simulink model "One_D_admittance_simulink"  (R2019b)
settings: Solver=ode45  StartTime=0.0  StopTime=50.0  RelTol=1e-4
model workspace (MAT data in the model file):
  k = Simulink.Parameter
  k.DataType = 'auto'
  k.Dimensions = [0 0]
  k_p = -0.125
libraries: simulink x1
settings Model: OrderedModelArguments=off  Creator=KEYUR  LastModifiedBy=KEYUR
settings DataIOCC: ExternalInput=[t, y]  InitialState=initi_x  LoadExternalInput=on

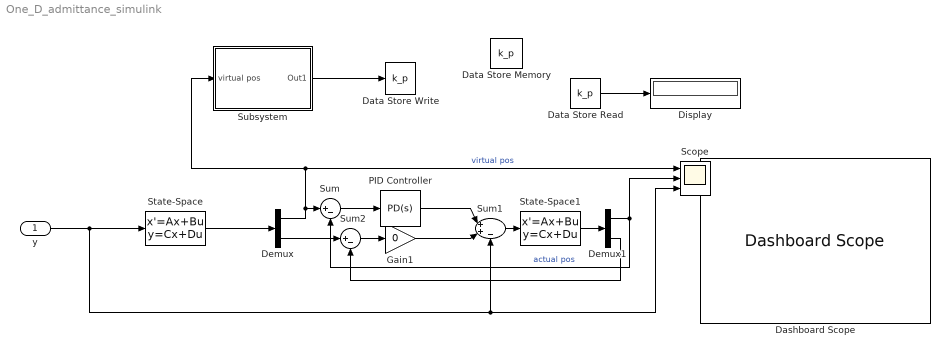
== system One_D_admittance_simulink ==
  y : Inport
  Dashboard Scope : DashboardScope  LegendPosition=Right
  Data Store Read : DataStoreRead  DataStoreName=k_p
  Data Store Write : DataStoreWrite  DataStoreName=k_p  DataStoreElements=k_p
  Data Store Memory : DataStoreMemory  DataStoreName=k_p  ReadBeforeWriteMsg=warning  WriteAfterWriteMsg=warning  WriteAfterReadMsg=warning  InitialValue=-10/40  VectorParams1D=off  ShowAdditionalParam=off  OutDataTypeStr=double
  Demux : Demux  Outputs=2
  Demux1 : Demux  Outputs=2
  Display : Display
  Gain1 : Gain  Gain=0
  PID Controller : simulink/Continuous/PID Controller  Controller=PD  Form=Parallel  TimeDomain=Continuous-time  SampleTime=-1  IntegratorMethod=Forward Euler  FilterMethod=Forward Euler  ControllerParametersSource=internal  P=85.3147223046163  I=6.85461887395414  D=89.8142135829374  UseFilter=on  N=224.237663795174  TunerSelectOption=Transfer Function Based (PID Tuner App)  InitialConditionSource=internal  InitialConditionForIntegrator=0  InitialConditionForFilter=0  DifferentiatorICPrevScaledInput=0  ExternalReset=none  TrackingMode=off  Kt=1  LimitOutput=off  UpperSaturationLimit=inf  LowerSaturationLimit=-inf  LinearizeAsGain=on  AntiWindupMode=none  Kb=1  POutMin=[]  POutMax=[]  IOutMin=[]  IOutMax=[]  DOutMin=[]  DOutMax=[]  NOutMin=[]  NOutMax=[]  SumOutMin=[]  SumOutMax=[]  SaturationOutMin=[]  SaturationOutMax=[]  PParamMin=[]  PParamMax=[]  IParamMin=[]  IParamMax=[]  DParamMin=[]  DParamMax=[]  NParamMin=[]  NParamMax=[]  KbParamMin=[]  KbParamMax=[]  KtParamMin=[]  KtParamMax=[]  KbOutMin=[]  KbOutMax=[]  KtOutMin=[]  KtOutMax=[]  IntegratorOutMin=[]  IntegratorOutMax=[]  FilterOutMin=[]  FilterOutMax=[]  SumI1OutMin=[]  SumI1OutMax=[]  SumI2OutMin=[]  SumI2OutMax=[]  SumI3OutMin=[]  SumI3OutMax=[]  SumI4OutMin=[]  SumI4OutMax=[]  SumDOutMin=[]  SumDOutMax=[]  DifferentiatorOutMin=[]  DifferentiatorOutMax=[]  FilterDiffOutCoefMin=[]  FilterDiffOutCoefMax=[]  ReciprocalOutMin=[]  ReciprocalOutMax=[]  SumDenOutMin=[]  SumDenOutMax=[]  SumNumOutMin=[]  SumNumOutMax=[]  DivideOutMin=[]  DivideOutMax=[]  IntegratorContinuousStateAttributes=''  IntegratorStateMustResolveToSignalObject=off  IntegratorRTWStateStorageClass=Auto  FilterContinuousStateAttributes=''  FilterStateMustResolveToSignalObject=off  FilterRTWStateStorageClass=Auto  ParallelPVariant=InternalParameters  IdealPVariant=Disabled  IVariant=Disabled  DVariant=InternalParameters  IntegratorVariant=Disabled  SatVariant=Disabled  AWVariant=Disabled  PCopyVariant=Disabled  TRVariant=Disabled  FdbkBlocksVariant=Forward  IdealPFdbkVariant=Disabled  SatFdbkVariant=Disabled  DerivativeFilterVariant=ContFilter  NVariant=InternalParameters  NCopyVariant=Disabled  FilterICVariant=InternalICsFilter  IntegratorICVariant=Disabled  ExternalResetVariant=Disabled  TRSumVariant=Passthrough  SumFdbkVariant=Disabled  SumVariant=Sum_PD
  Scope : Scope  NumInputPorts=3
  State-Space : StateSpace  A=[0,1 ; k_p, -10/40]  B=[0 ; 1/40]  C=[1 0;0 1]  D=[0 ; 0]  InitialCondition=0
  State-Space1 : StateSpace  A=[0,1 ; 0, -20/100]  B=[0 ; 1/100]  C=[1 0;0 1]  D=[0;0]  InitialCondition=0
  Subsystem : Subsystem
  Sum : Sum  Inputs=|+-
  Sum1 : Sum  Inputs=|++-
  Sum2 : Sum  Inputs=|+-
  wires:
  Sum1/1 -> State-Space1/1
  State-Space/1 -> Demux/1
  Demux/1 -> Subsystem/1(virtual pos), Scope/1, Sum/1  "virtual pos"
  State-Space1/1 -> Demux1/1
  Demux1/1 -> Sum/2, Scope/2  "actual pos"
  Demux/2 -> Sum2/1
  Demux1/2 -> Sum2/2
  Sum/1 -> PID Controller/1
  Sum2/1 -> Gain1/1
  Gain1/1 -> Sum1/2
  PID Controller/1 -> Sum1/1
  y/1 -> Scope/3, Sum1/3, State-Space/1
  Subsystem/1(Out1) -> Data Store Write/1
  Data Store Read/1 -> Display/1

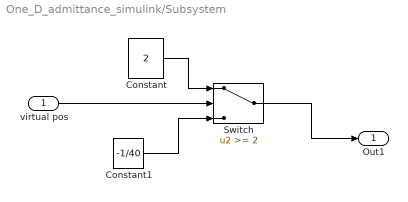
== system One_D_admittance_simulink/Subsystem ==
  virtual pos : Inport
  Constant : Constant  Value=2
  Constant1 : Constant  Value=-1/40
  Switch : Switch  Threshold=2
  Out1 : Outport
  wires:
  Constant/1 -> Switch/1
  Constant1/1 -> Switch/3
  virtual pos/1 -> Switch/2
  Switch/1 -> Out1/1
